simulink subsystem "Odometria"  (R2024b)
settings: Solver=VariableStepAuto  StartTime=0.0  StopTime=10.0  RelTol=1e-3
undefined symbols (not defined in the file): DiscIntNeverNeededParam
settings Model: Creator=Chenfu  LastModifiedBy=Chenfu

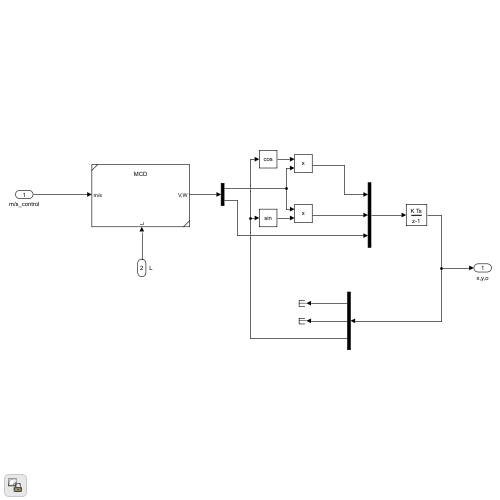
[thumbnail: Simulink's stored preview of the top-level diagram]
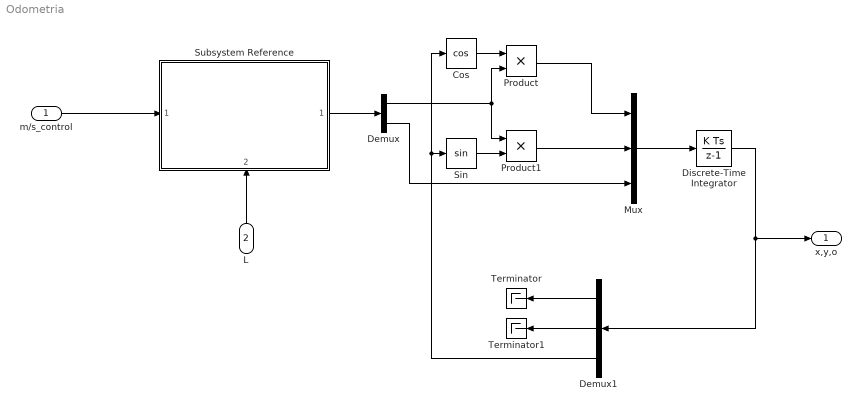
== system Odometria ==
  m/s_control : Inport
  L : Inport  Port=2
  Cos : Trigonometry  Operator=cos
  Demux : Demux  Outputs=2
  Demux1 : Demux  Outputs=3
  Discrete-Time Integrator : DiscreteIntegrator  SampleTime=-1  ICPrevOutput=DiscIntNeverNeededParam  ICPrevScaledInput=DiscIntNeverNeededParam
  Mux : Mux  Inputs=3
  Product : Product
  Product1 : Product
  Sin : Trigonometry
  Subsystem Reference : Subsystem  ReferencedSubsystem=MCD
      settings: PortSchema="{\"entries\":[{\"content\":{\"sides\":[{\"content\":{\"connectorIds\":[\"In1\"]},\"type\":\"ConnectorPlacement.EquallySpacedRectSide\",\"uuid\":\"34ece06b-3d35-4367-a5d8-77f3d20531fe\"},{\"content\":{\"connectorIds\":[\"Out1\"],\"side\":\"RIGHT\"},\"type\":\"ConnectorPlacement.EquallySpacedRectSide\",\"uuid\":\"f174795e-9c72-4515-a183-1488b74a6279\"},{\"content\":{\"side\":\"TOP\"},\"type\":\"ConnectorPlacement.EquallySpacedRectSide\",\"uuid\":\"48fa7938-9ff0-440f-a4dd-a4ef578a1135\"},{\"content\":{\"connectorIds\":[\"In2\"],\"side\":\"BOTTOM\"},\"type\":\"ConnectorPlacement.EquallySpacedRectSide\",\"uuid\":\"0103d935-d181-40ca-a9d2-1122bf328f0b\"}]},\"type\":\"ConnectorPlacement.EquallySpacedConnector\",\"uuid\":\"0da01e04-506c-4b41-953a-19be5e9a17e2\"}],\"packageUris\":[\"http://schema.mathworks.com/mf0/Connector/R2020b\"],\"version\":\"1.0\"}"
  Terminator : Terminator
  Terminator1 : Terminator
  x,y,o : Outport
  wires:
  m/s_control/1 -> Subsystem Reference/1
  L/1 -> Subsystem Reference/2
  Subsystem Reference/1 -> Demux/1
  Cos/1 -> Product/1
  Sin/1 -> Product1/2
  Demux1/1 -> Terminator/1
  Demux1/2 -> Terminator1/1
  Demux1/3 -> Sin/1, Cos/1
  Product/1 -> Mux/1
  Demux/1 -> Product/2, Product1/1
  Product1/1 -> Mux/2
  Demux/2 -> Mux/3
  Mux/1 -> Discrete-Time Integrator/1
  Discrete-Time Integrator/1 -> x,y,o/1, Demux1/1
